simulink model "3DOF_Nonlinear_Simulink_Model"  (R2019b)
settings: Solver=VariableStepAuto  StartTime=0.0  StopTime=9.25  RelTol=1e-3
values from neighbouring files (symbols this model uses):
  epsf = 0    [Linear_3DOF_With_Roll.m]    (also in Nonlinear_3DOF_With_Roll.m = 0.04)
  epsr = -0.03    [Linear_3DOF_With_Roll.m]    (also in Nonlinear_3DOF_With_Roll.m = 0.04)
  fo_SI = fo*4.448    (= 4448)    [Nonlinear_3DOF_With_Roll.m]
  h1_SI = h1*0.305    (= 0.1525)    [Linear_3DOF_With_Roll.m]    (also in Nonlinear_3DOF_With_Roll.m)
  hr_SI = hcg_SI-h1_SI    (= 0.2135)    [Linear_3DOF_With_Roll.m]    (also in Nonlinear_3DOF_With_Roll.m)
  Iz_SI = Iz/23.73036    (= 1685.60443247)    [Linear_2DOF_Bicycle_Model.m]    (also in Linear_3DOF_With_Roll.m; NonLinear_2DOF.m; Nonlinear_3DOF_With_Roll.m)
  lf_SI = 3.5*0.305    (= 1.0675)    [Linear_2DOF_Bicycle_Model.m]    (also in Linear_3DOF_With_Roll.m; NonLinear_2DOF.m; Nonlinear_3DOF_With_Roll.m)
  lr_SI = 4.5*0.305    (= 1.3725)    [Linear_2DOF_Bicycle_Model.m]    (also in Linear_3DOF_With_Roll.m; NonLinear_2DOF.m; Nonlinear_3DOF_With_Roll.m)
  m_SI = 3000*0.453592    (= 1360.776)    [Linear_2DOF_Bicycle_Model.m]    (also in Linear_3DOF_With_Roll.m; NonLinear_2DOF.m; Nonlinear_3DOF_With_Roll.m)
  roll_dampingf = 1*i^2    [Nonlinear_3DOF_With_Roll.m]
  roll_dampingr = 3*i^2    [Nonlinear_3DOF_With_Roll.m]
  roll_stiffnessf = 10*i^2    [Nonlinear_3DOF_With_Roll.m]
  roll_stiffnessr = 60*i^2    [Nonlinear_3DOF_With_Roll.m]
  t_SI = 6*0.305    (= 1.83)    [Nonlinear_3DOF_With_Roll.m]
  Wf_SI = mf_SI*9.81    (= 7508.932065)    [Nonlinear_3DOF_With_Roll.m]
  Wr_SI = mr_SI*9.81    (= 5840.280495)    [Nonlinear_3DOF_With_Roll.m]
undefined symbols (not defined in the file or in its folder): vxs
libraries: simulink x6, simulink_extras x1
settings Model: Creator=Jad Yahya  LastModifiedBy=Jad Yahya

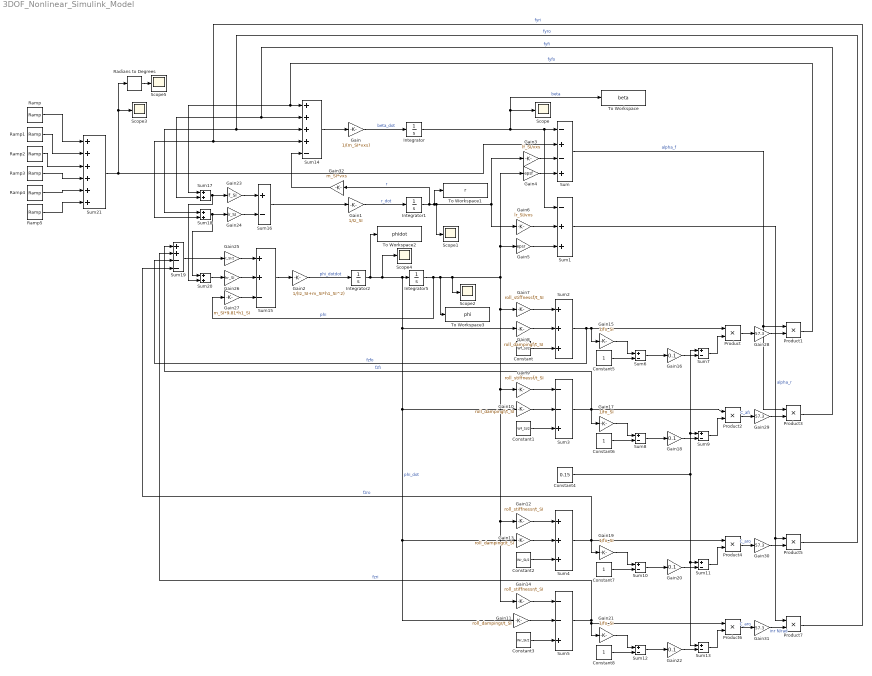
== system 3DOF_Nonlinear_Simulink_Model ==
  Constant : Constant  Value=Wf_SI/2
  Constant1 : Constant  Value=Wf_SI/2
  Constant2 : Constant  Value=Wr_SI/2
  Constant3 : Constant  Value=Wr_SI/2
  Constant4 : Constant  Value=0.15
  Constant{5..8} (4 alike) : Constant
  Gain : Gain  Gain=1/(m_SI*vxs)
  Gain1 : Gain  Gain=1/Iz_SI
  Gain10 : Gain  Gain=roll_dampingf/t_SI
  Gain11 : Gain  Gain=roll_dampingr/t_SI
  Gain12 : Gain  Gain=roll_stiffnessr/t_SI
  Gain13 : Gain  Gain=roll_dampingr/t_SI
  Gain14 : Gain  Gain=roll_stiffnessr/t_SI
  Gain{15,17,19,21} (4 alike) : Gain  Gain=1/fo_SI
  Gain{16,18,20,22} (4 alike) : Gain  Gain=0.1
  Gain2 : Gain  Gain=1/(Iz_SI+m_SI*h1_SI^2)
  Gain23 : Gain  Gain=lf_SI
  Gain24 : Gain  Gain=lr_SI
  Gain25 : Gain  Gain=t_SI/2
  Gain26 : Gain  Gain=hr_SI
  Gain27 : Gain  Gain=m_SI*9.81*h1_SI
  Gain{28..31} (4 alike) : Gain  Gain=57.3
  Gain3 : Gain  Gain=lf_SI/vxs
  Gain32 : Gain  Gain=m_SI*vxs
  Gain4 : Gain  Gain=epsf
  Gain5 : Gain  Gain=epsr
  Gain6 : Gain  Gain=lr_SI/vxs
  Gain7 : Gain  Gain=roll_stiffnessf/t_SI
  Gain8 : Gain  Gain=roll_dampingf/t_SI
  Gain9 : Gain  Gain=roll_stiffnessf/t_SI
  Integrator{,1..2,5} (4 alike) : Integrator
  Product{,1..7} (8 alike) : Product
  Radians to Degrees : simulink_extras/Transformations/Radians to Degrees
  Ramp : simulink/Sources/Ramp  slope=720/57.3  start=0  InitialOutput=0
  Ramp1 : simulink/Sources/Ramp  slope=-720/57.3  start=0.0625  InitialOutput=0
  Ramp2 : simulink/Sources/Ramp  slope=-720/57.3  start=3.0625  InitialOutput=0
  Ramp3 : simulink/Sources/Ramp  slope=+720/57.3  start=3.1875  InitialOutput=0
  Ramp4 : simulink/Sources/Ramp  slope=+720/57.3  start=6.1875  InitialOutput=0
  Ramp5 : simulink/Sources/Ramp  slope=-720/57.3  start=6.25  InitialOutput=0
  Scope{,1..5} (6 alike) : Scope
  Sum : Sum  Inputs=-+-+
  Sum1 : Sum  Inputs=-++
  Sum{6..13,16} (9 alike) : Sum  Inputs=+-
  Sum14 : Sum  Inputs=++++-
  Sum15 : Sum  Inputs=++-
  Sum17 : Sum
  Sum18 : Sum
  Sum19 : Sum  Inputs=++--
  Sum2 : Sum  Inputs=+++
  Sum20 : Sum
  Sum21 : Sum  Inputs=++++++
  Sum3 : Sum  Inputs=--+
  Sum4 : Sum  Inputs=+++
  Sum5 : Sum  Inputs=--+
  To Workspace : ToWorkspace  VariableName=beta  SampleTime=-1
  To Workspace1 : ToWorkspace  VariableName=r  SampleTime=-1
  To Workspace2 : ToWorkspace  VariableName=phidot  SampleTime=-1
  To Workspace3 : ToWorkspace  VariableName=phi  SampleTime=-1
  wires:
  Gain/1 -> Integrator/1  "beta_dot"
  Gain1/1 -> Integrator1/1  "r_dot"
  Gain2/1 -> Integrator2/1  "phi_dotdot"
  Integrator2/1 -> To Workspace2/1, Scope4/1, Gain11/1, Gain13/1, Gain10/1, Gain8/1, Integrator5/1  "phi_dot"
  Integrator1/1 -> Gain32/1, To Workspace1/1, Scope1/1, Gain6/1, Gain3/1  "r"
  Integrator/1 -> To Workspace/1, Scope/1, Sum/1, Sum1/1  "beta"
  Sum21/1 -> Radians to Degrees/1, Scope3/1, Sum/2
  Gain3/1 -> Sum/3
  Integrator5/1 -> Gain27/1, To Workspace3/1, Scope2/1, Gain12/1, Gain14/1, Gain9/1, Gain7/1, Gain5/1, Gain4/1  "phi"
  Gain4/1 -> Sum/4
  Gain5/1 -> Sum1/3
  Gain6/1 -> Sum1/2
  Constant/1 -> Sum2/3
  Gain7/1 -> Sum2/1
  Gain8/1 -> Sum2/2
  Gain10/1 -> Sum3/2
  Gain9/1 -> Sum3/1
  Constant1/1 -> Sum3/3
  Constant3/1 -> Sum5/3
  Gain14/1 -> Sum5/1
  Gain11/1 -> Sum5/2
  Gain13/1 -> Sum4/2
  Gain12/1 -> Sum4/1
  Constant2/1 -> Sum4/3
  Sum2/1 -> Gain15/1, Product/1, Sum19/3  "fzfo"
  Gain15/1 -> Sum6/1
  Constant5/1 -> Sum6/2
  Sum6/1 -> Gain16/1
  Gain16/1 -> Sum7/2
  Sum7/1 -> Product/2
  Product/1 -> Gain28/1
  Sum/1 -> Product3/1, Product1/1  "alpha_f"
  Product2/1 -> Gain29/1  "C_afi"
  Sum9/1 -> Product2/2
  Gain18/1 -> Sum9/2
  Sum8/1 -> Gain18/1
  Constant6/1 -> Sum8/2
  Gain17/1 -> Sum8/1
  Sum3/1 -> Gain17/1, Product2/1, Sum19/1  "fzfi"
  Sum4/1 -> Gain19/1, Product4/1, Sum19/4  "fzro"
  Gain19/1 -> Sum10/1
  Sum10/1 -> Gain20/1
  Gain20/1 -> Sum11/2
  Sum11/1 -> Product4/2
  Product4/1 -> Gain30/1  "C_aro"
  Constant4/1 -> Sum13/1, Sum11/1, Sum9/1, Sum7/1
  Constant7/1 -> Sum10/2
  Sum1/1 -> Product7/1, Product5/1  "alpha_r"
  Constant8/1 -> Sum12/2
  Product6/1 -> Gain31/1  "C_aro"
  Sum13/1 -> Product6/2
  Gain22/1 -> Sum13/2
  Sum12/1 -> Gain22/1
  Gain21/1 -> Sum12/1
  Sum5/1 -> Gain21/1, Product6/1, Sum19/2  "fzri"
  Sum14/1 -> Gain/1
  Product1/1 -> Sum17/1, Sum14/1  "fyfo"
  Product3/1 -> Sum17/2, Sum14/2  "fyfi"
  Product5/1 -> Sum18/1, Sum14/3  "fyro"
  Product7/1 -> Sum18/2, Sum14/4  "fyri"
  Sum15/1 -> Gain2/1
  Sum16/1 -> Gain1/1
  Gain23/1 -> Sum16/1
  Sum17/1 -> Sum20/2, Gain23/1
  Sum18/1 -> Sum20/1, Gain24/1
  Gain24/1 -> Sum16/2
  Sum19/1 -> Gain25/1
  Gain25/1 -> Sum15/1
  Gain26/1 -> Sum15/2
  Sum20/1 -> Gain26/1
  Gain27/1 -> Sum15/3
  Ramp/1 -> Sum21/1
  Ramp1/1 -> Sum21/2
  Ramp2/1 -> Sum21/3
  Ramp3/1 -> Sum21/4
  Ramp4/1 -> Sum21/5
  Ramp5/1 -> Sum21/6
  Radians to Degrees/1 -> Scope5/1
  Gain28/1 -> Product1/2
  Gain29/1 -> Product3/2
  Gain30/1 -> Product5/2
  Gain31/1 -> Product7/2  "inr N/rad"
  Gain32/1 -> Sum14/5
